simulink model "Z_trajectory_SMC_with_functions"  (R2018b)
settings: Solver=FixedStepAuto  StartTime=0.0  StopTime=10.0  RelTol=1e-3  EnableMultiTasking=on
undefined symbols (not defined in the file or in its folder): dev, Main, pwm_output0
libraries: px4Sensorslib x3, px4lib x1, px4uORBlib x1
settings Model: ExtModeTrigDuration=10  Creator=Tejas Rajopadhye  LastModifiedBy=Tejas Rajopadhye
settings SolverCC: PositivePriorityOrder=on  AutoInsertRateTranBlk=on
settings OptimizationCC: EnhancedBackFolding=on  PassReuseOutputArgsAs=Individual arguments  MaxStackSize=64  OptimizeBlockOrder=speed  DifferentSizesBufferReuse=on  OptimizationCustomize=off
settings DebuggingCC: ParameterTunabilityLossMsg=error
settings HardwareCC: ProdBitPerPointer=32  ProdBitPerSizeT=32  ProdBitPerPtrDiffT=32  ProdLargestAtomicInteger=Long  ProdLargestAtomicFloat=Double  ProdWordSize=32  ProdLongLongMode=on  ProdHWDeviceType=ARM Compatible->ARM Cortex
settings SFSimCC: MATLABDynamicMemAlloc=off
settings RTWCC: SystemTargetFile=ert.tlc  HardwareBoard=PX4 Pixhawk 4  TLCOptions="-aInlineSetEventsForThisBaseRateFcn=TLC_FALSE -aSuppressMultiTaskScheduler=TLC_FALSE  -aRateBasedStepFcn=0"  TemplateMakefile=ert_default_tmf  GenerateReport=on  Toolchain=GNU Tools for PX4 Autopilots  IncludeHyperlinkInReport=on  LaunchReport=on  TargetLang=C++  GenerateTraceInfo=on  GenerateTraceReport=on  GenerateTraceReportSl=on  GenerateTraceReportSf=on  GenerateTraceReportEml=on
settings CodeAppCC: ForceParamTrailComments=on  IgnoreCustomStorageClasses=off  OperatorAnnotations=on  SimulinkDataObjDesc=on  SFDataObjDesc=on  InsertBlockDesc=on

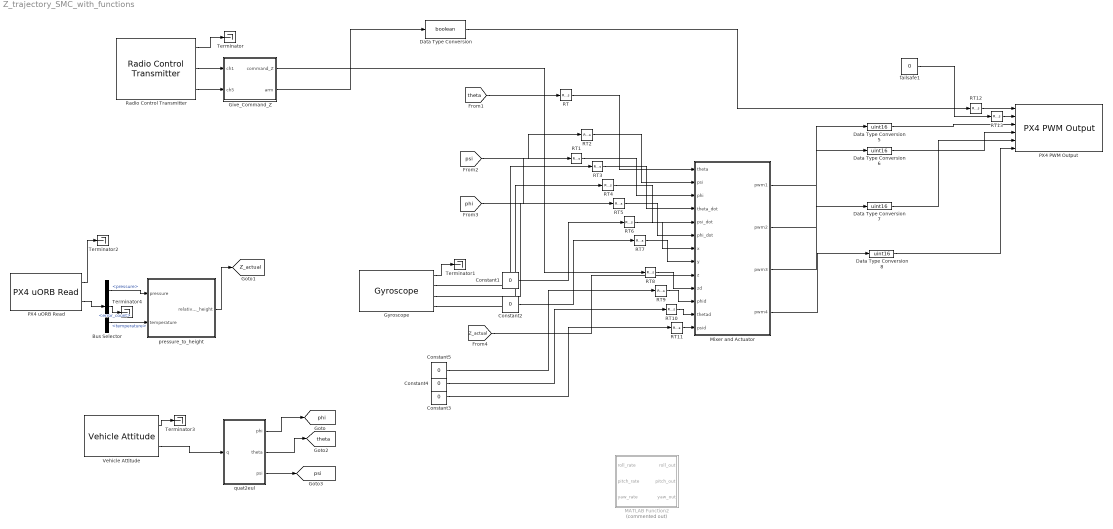
== system Z_trajectory_SMC_with_functions ==
  Bus Selector : BusSelector  OutputSignals=pressure,error_count,temperature
  Constant{1..5} (5 alike) : Constant  Value=0  OutDataTypeStr=uint16  SampleTime=1/250
  Data Type Conversion : DataTypeConversion  OutDataTypeStr=boolean
  Data Type Conversion{5..8} (4 alike) : DataTypeConversion  OutDataTypeStr=uint16
  Give_Command_Z : MATLAB Function  TreatAsAtomicUnit=on
  Gyroscope : px4Sensorslib/Gyroscope  uorbTimeStamp=off  BlockingMode=off  BlockTimeout=1e-3  sampleTime=1/250
      settings: SourceProductName=Embedded Coder Support Package for PX4 Autopilots
  MATLAB Function2 : MATLAB Function  Commented=on  TreatAsAtomicUnit=on
  Mixer and Actuator : MATLAB Function  TreatAsAtomicUnit=on
  PX4 PWM Output : px4lib/PX4 PWM Output  pwmDevice=Main (/dev/pwm_output0)  pwmChannel1_=on  pwmChannel2_=on  pwmChannel3_=on  pwmChannel4_=on  pwmChannel5_=off  pwmChannel6_=off  pwmChannel7_=off  pwmChannel8_=off  forceTerminateFailsafe=off  outputErrorStatus=off
      settings: SourceProductName=Embedded Coder Support Package for PX4 Autopilots  SourceProductBaseCode=PX4AUTOPILOTS
  PX4 uORB Read : px4uORBlib/PX4 uORB Read  uORBTopic=sensor_baro  sampleTime=-1  BlockingMode=off  BlockTimeout=1e-3
      settings: SourceProductName=Embedded Coder Support Package for PX4 Autopilots
  RT{,1..13} (14 alike) : RateTransition  OutPortSampleTime=0.002
  Radio Control Transmitter : px4Sensorslib/Radio Control Transmitter  channel1=on  channel2=off  channel3=off  channel4=off  channel5=on  channel6=off  channel7=off  channel8=off  channel_count=off  rssi=off  rc_input_source=off  timestamp_last_signal=off  time_stamp=off  sampleTime=1/250  BlockingMode=off  BlockTimeout=5
      settings: SourceProductName=Embedded Coder Support Package for PX4 Autopilots
  Terminator{,1..4} (5 alike) : Terminator
  Vehicle Attitude : px4Sensorslib/Vehicle Attitude  rollRate=off  pitchRate=off  yawRate=off  quaternion=on  uorbTimeStamp=off  BlockingMode=off  BlockTimeout=0.001  sampleTime=1/250
      settings: SourceProductName=Embedded Coder Support Package for PX4 Autopilots
  failsafe1 : Constant  Value=0  OutDataTypeStr=boolean  SampleTime=0.01
  pressure_to_height : MATLAB Function  TreatAsAtomicUnit=on
  quat2eul : MATLAB Function  TreatAsAtomicUnit=on
  tag scope: Z_actual=global, phi=global, psi=global, theta=global
  wires:
  Radio Control Transmitter/1 -> Terminator/1
  Radio Control Transmitter/2 -> Give_Command_Z/1(ch1)
  Mixer and Actuator/1(pwm1) -> Data Type Conversion5/1
  Mixer and Actuator/2(pwm2) -> Data Type Conversion6/1
  Mixer and Actuator/3(pwm3) -> Data Type Conversion7/1
  Mixer and Actuator/4(pwm4) -> Data Type Conversion8/1
  Radio Control Transmitter/3 -> Give_Command_Z/2(ch5)
  Give_Command_Z/2(arm) -> Data Type Conversion/1
  failsafe1/1 -> RT13/1
  Data Type Conversion5/1 -> PX4 PWM Output/3
  Data Type Conversion8/1 -> PX4 PWM Output/6
  Data Type Conversion6/1 -> PX4 PWM Output/4
  Data Type Conversion7/1 -> PX4 PWM Output/5
  Vehicle Attitude/1 -> Terminator3/1
  Vehicle Attitude/2 -> quat2eul/1(q)
  quat2eul/3(psi) -> [psi]
  quat2eul/2(theta) -> [theta]
  quat2eul/1(phi) -> [phi]
  PX4 uORB Read/2 -> Bus Selector/1
  PX4 uORB Read/1 -> Terminator2/1
  Bus Selector/2 -> Terminator4/1  "<error_count>"
  Bus Selector/1 -> pressure_to_height/1(pressure)  "<pressure>"
  Bus Selector/3 -> pressure_to_height/2(temperature)  "<temperature>"
  pressure_to_height/1(relative_height) -> [Z_actual]
  Data Type Conversion/1 -> RT12/1
  [theta] -> RT/1
  [psi] -> RT2/1
  [phi] -> RT1/1
  Gyroscope/1 -> Terminator1/1
  Gyroscope/2 -> RT3/1
  Gyroscope/4 -> RT4/1
  Gyroscope/3 -> RT5/1
  Give_Command_Z/1(command_Z) -> RT8/1
  Constant3/1 -> RT11/1
  Constant5/1 -> RT9/1
  [Z_actual] -> Mixer and Actuator/9(z)
  Constant4/1 -> RT10/1
  Constant1/1 -> RT6/1
  Constant2/1 -> RT7/1
  RT/1 -> Mixer and Actuator/1(theta)
  RT1/1 -> Mixer and Actuator/3(phi)
  RT2/1 -> Mixer and Actuator/2(psi)
  RT3/1 -> Mixer and Actuator/4(theta_dot)
  RT4/1 -> Mixer and Actuator/5(psi_dot)
  RT5/1 -> Mixer and Actuator/6(phi_dot)
  RT6/1 -> Mixer and Actuator/7(x)
  RT7/1 -> Mixer and Actuator/8(y)
  RT8/1 -> Mixer and Actuator/10(zd)
  RT9/1 -> Mixer and Actuator/11(phid)
  RT10/1 -> Mixer and Actuator/12(thetad)
  RT11/1 -> Mixer and Actuator/13(psid)
  RT12/1 -> PX4 PWM Output/1
  RT13/1 -> PX4 PWM Output/2

== matlab function Z_trajectory_SMC_with_functions/Give_Command_Z ==
  data: ch1 input; command_Z output; ch5 input; arm output
function [command_Z, arm] = Commands(ch1, ch5)
ch1 = single(ch1);
command_Z = (ch1 - 1000)/100; %for z trajecctory from 0 to 10m
if (ch5 > single(1500))
    arm = true;
else
    arm = false;
end

== matlab function Z_trajectory_SMC_with_functions/pressure_to_height ==
  data: pressure input; relative_height output; temperature input
function relative_height = covert_pressure_to_height(pressure, temperature)
R = single(287);
g = single(9.81);
temperature = temperature + single(273.15); %convert to kelvin from degrees

persistent itr;
if isempty(itr)
    itr = 0;
end

persistent init_pressure;
if isempty(init_pressure)
    init_pressure = single(944.77);
end

if (itr == 0)
    initial_pressure = pressure;
    itr = itr + 1;
else
    initial_pressure = single(init_pressure);
end

if (isreal(log(pressure/initial_pressure)))
    log_value = log(pressure/initial_pressure);
else
    log_value = 0;
end

init_pressure = single(initial_pressure);

relative_height = single(((R*temperature)/g)*log_value);

== matlab function Z_trajectory_SMC_with_functions/MATLAB Function2 ==
  data: roll_rate input; roll_out output; pitch_rate input; yaw_rate input; pitch_out output; yaw_out output
function [roll_out, pitch_out, yaw_out] = rates_to_actual(roll_rate, pitch_rate, yaw_rate)
persistent roll;
persistent pitch;
persistent yaw;
if isempty(roll || pitch || yaw)
    roll = 0;
    pitch = 0;
    yaw = 0;
end
    
integral_time = single(0.004);

roll = roll + roll_rate*integral_time;
pitch = pitch + pitch_rate*integral_time;
yaw = yaw + yaw_rate*integral_time;

roll_out = roll;
pitch_out = pitch;
yaw_out = yaw;

== matlab function Z_trajectory_SMC_with_functions/Mixer and Actuator ==
  data: theta input; pwm1 output; psi input; phi input; theta_dot input; psi_dot input; phi_dot input; x input; y input; z input; zd input; phid input; thetad input; psid input; pwm2 output; pwm3 output; pwm4 output
function [pwm1,pwm2,pwm3,pwm4] = SMC_block(theta, psi , phi, theta_dot, psi_dot, phi_dot, x, y ,z, zd, phid, thetad, psid)
% int xd;  %Define this later
% int yd; 

%Constants / Controller constants

a1 = single(0.8);
a2 = single(0.8);
a3 = single(0.9);
a4 = single(7);
a5 = single(7);
a6 = single(5);

k1 = single(1.98);
k2 = single(1.98);
k3 = single(2.78);
k4 = single(5.25);
k5 = single(5.25);
k6 = single(2.75);

l1 = single(0.9);
l2 = single(0.9);
l3 = single(1.25);
l4 = single(3.5);
l5 = single(3.5);
l6 = single(1.8);


zd_dot = single(0);
zd_dot_dot = single(0);
persistent phidprev phidrecent thetadprev thetadrecent phid_dotprev thetad_dotprev phid_dot_dot thetad_dot_dot;

if (isempty(phidprev))
    phidprev = single(0);
end
if (isempty(phidrecent))
    phidrecent = single(0);
end

if (isempty(thetadprev))
    thetadprev = single(0);
end

if (isempty(thetadrecent))
    thetadrecent = single(0);
end

if (isempty(phid_dotprev))
    phid_dotprev = single(0);
end

if (isempty(thetad_dotprev))
    thetad_dotprev = single(0);
end

if (isempty(phid_dot_dot))
    phid_dot_dot = single(0);
end

if (isempty(thetad_dot_dot))
    thetad_dot_dot = single(0);
end

psid_dot_dot = single(0);
psid_dot = single(0);


Ix = single(0.047);
Iy = single(0.047);
Iz = single(0.094);
m = single(0.93);

g = single(9.81);
L = single(0.225);

ct = single(0.0984);    % Values from doc
cm = single(0.00679);   % Values from doc
 
t = 0.004;   %Updated time step to the base rate of model
% Above are the desired values to be taken as input from the user
% Take all the current values from the gps and gyro etc
% variables xd_dot are desired rate of changes in the setpoint. Current we
% set it as zero
% calculate cos of theta and phi
% Assign all the values from a1 to a6, k1 to k6 and l1 to l6
% Define constants like ct, cm and L

% Values of phid and thetad will be iteratively modified based on ux and uy
% values 
% Thus phid and thetad will be non zero and will have to be calculated

% set phid and thetad as zero initially (please calculate its derivative
% somewhere, i cant figure out where to calcualte it

% phid_dot = (phidrecent - phidprev)/t;
% thetad_dot = (thetadrecent - thetadprev)/t;

phid_dot = single(0);
thetad_dot = single(0);

% phid_dot_dot = (phid_dot - phid_dotprev)/t;
% thetad_dot_dot = (thetad_dot - thetad_dotprev)/t;

phid_dot_dot = single(0);
thetad_dot_dot = single(0);

% phid_dotprev = phid_dot; % assign initial values of both   equal to zero
% thetad_dotprev = thetad_dot; % assign initial values of both   equal to zero

phid_dotprev = single(0);
thetad_dotprev = single(0);

phid = single(0);
thetad = single(0);
psid = single(0);
zprev = single(0);

% s1 = (x-xprev)/t - xd_dot + a1*(x-xd); % t is timestep
% s2 = (y-yprev)/t - yd_dot + a2*(y-yd);
s3 = (z-zprev)/t - zd_dot + a3*(z-zd);
s4 = phi_dot- phid_dot + a4*(phi-phid);
s5 = theta_dot - thetad_dot + a5*(theta-thetad);
s6 = psi_dot - psid_dot + a6*(psi-psid);

% if s1 > 0 
%     sign_s1 = 1;
% else
%     sign_s1 = -1;
% end
% 
% if s2 > 0 
%     sign_s2 = 1;
% else
%     sign_s2 = -1;
% end

if s3 > 0 
    sign_s3 = 1;
else
    sign_s3 = -1;
end

if s4 > 0 
    sign_s4 = 1;
else
    sign_s4 = -1;
end

if s5 > 0 
    sign_s5 = 1;
else
    sign_s5 = -1;
end

if s6 > 0 
    sign_s6 = 1;
else
    sign_s6 = -1;
end

u4 = (m*g/(cos(phi) * cos(theta)))*(zd_dot_dot - a3*((z-zprev)/t - zd_dot) - k3*sign_s3 - l3*s3);
% ux = (m/u4)*(xd_dot_dot - a1*((x-xprev)/t - xd_dot) - k1*sign_s1 - l1*s1);
% uy = (m/u4)*(yd_dot_dot - a2*((y-yprev)/t - yd_dot) - k2*sign_s2 - l2*s2);
u1 = Ix * (phid_dot_dot - a4*(phi_dot - phid_dot) - k4*sign_s4 - l4*s4 - ((Iy-Iz)/Ix)*(theta_dot)*(psi_dot));
u2 = Iy * (thetad_dot_dot - a5*(theta_dot - thetad_dot) - k5*sign_s5 - l5*s5 - ((Iz-Ix)/Iy)*(phi_dot)*(psi_dot));
u3 = Iz * (psid_dot_dot - a6*(psi_dot - psid_dot) - k6*sign_s6 - l6*s6 - ((Ix-Iy)/Iz)*(phi_dot)*(theta_dot));

zprev = z;
% phidprev = phidrecent; % assign initial values of both   equal to zero
% thetadprev = thetadrecent; % assign initial values of both   equal to zero


% calculate sine and cosines here
% and take sine inverse
% phid = asin(sin_psi * ux + cos_psi * uy);
% thetad = asin((cos_psi * ux + sin_psi * uy)/cos_phid);

% phidrecent = phid;
% thetadrecent = thetad;


% Finding square of speed of motors from the thrusts
w1_sq = u4/(4*ct) - u3/(4*cm) - u2/(2*L*ct);
w2_sq = u4/(4*ct) + u3/(4*cm) - u1/(2*L*ct);
w3_sq = u4/(4*ct) - u3/(4*cm) + u2/(2*L*ct);
w4_sq = u4/(4*ct) + u3/(4*cm) + u1/(2*L*ct);

w1 = sqrt(w1_sq);
w2 = sqrt(w2_sq);
w3 = sqrt(w3_sq);
w4 = sqrt(w4_sq);

pwm1 = (w1*2.0e-3)/11000;
pwm2 = (w2*2.0e-3)/11000;
pwm3 = (w3*2.0e-3)/11000;
pwm4 = (w4*2.0e-3)/11000;

if (pwm1 < single(900) || pwm2 < single(900) || pwm3 < single(900) || pwm4 < single(900))
    pwm1 = single(900);
    pwm2 = single(900);
    pwm3 = single(900);
    pwm4 = single(900);
end

== matlab function Z_trajectory_SMC_with_functions/quat2eul ==
  data: q input; phi output; theta output; psi output
function [phi,theta,psi] = quat2eul(q)
% Conversion from Quaternion to Euler angles based on the PX4 Firmware
% v1.6.5 release.
% 
% Quaternion -> DCM -> Euler Angles
% INPUT:
%   q: Quaternion vector of the format: (a + bi + cj + dk)
% OUTPUT:
%   [phi,theta,psi]: Euler angles in radians.
% 
 
    a = q(1);
    b = q(2);
    c = q(3);
    d = q(4);

    aSq = a*a;
    bSq = b*b;
    cSq = c*c;
    dSq = d*d;

    d_pi2 = pi/2;

    % quaternion_to_dcm
    dcm00 = aSq + bSq - cSq - dSq;
    % dcm01 = 2*(b*c - a*d);
    dcm02 = 2*(a*c + b*d);
    dcm10 = 2*(b*c + a*d);
    % dcm11 = aSq - bSq + cSq - dSq;
    dcm12 = 2*(c*d - a*b);
    dcm20 = 2*(b*d - a*c);
    dcm21 = 2*(a*b + c*d);
    dcm22 = aSq - bSq - cSq + dSq;

    % dcm_to_euler
    theta = asin(-dcm20);
    if abs(theta - d_pi2) < 1.0e-3
        phi = single(0.0);
        psi = atan2(dcm12, dcm02);
    elseif abs(theta + d_pi2) < 1.0e-3
        phi = single(0.0);
        psi = atan2(-dcm12, -dcm02);
    else
        phi = atan2(dcm21, dcm22);
        psi = atan2(dcm10, dcm00);
    end

end
